simulink model "sampleModel1939"  (R2023a)
settings: Solver=VariableStepAuto  StartTime=0.0  StopTime=10.0  RelTol=1e-3
libraries: hdlsllib x3, simulink x1
settings Model: Creator=user1  LastModifiedBy=user1

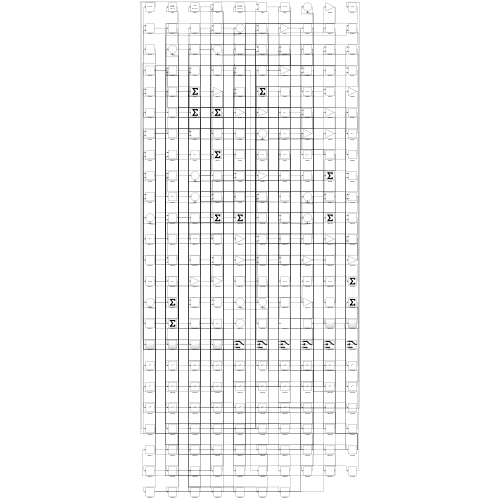
[thumbnail: Simulink's stored preview of the top-level diagram]
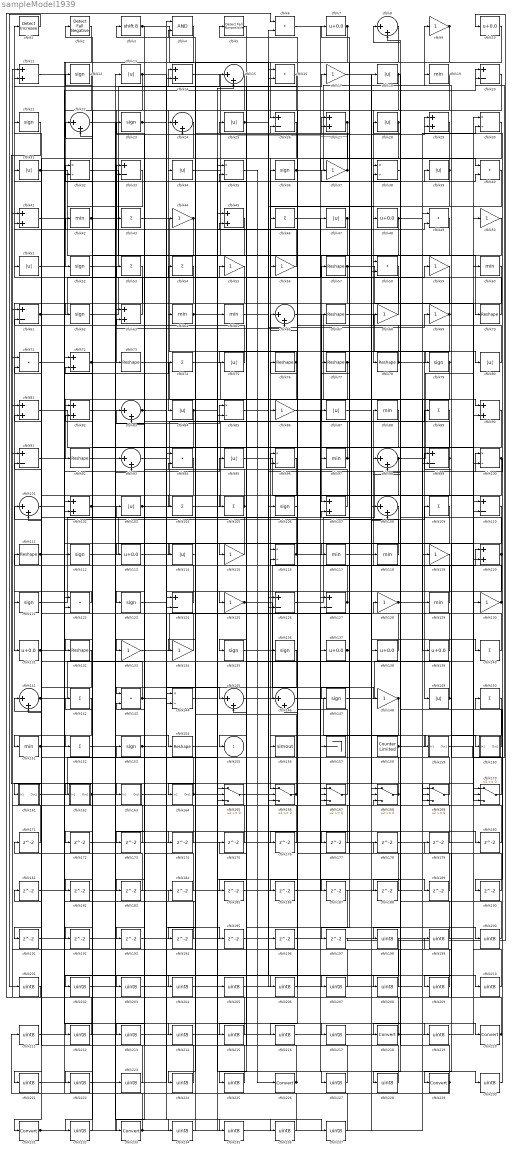
== system sampleModel1939 ==
  cfblk1 : simulink/Logic and Bit Operations/Detect Increase  vinit=0.0  OutDataTypeStr=boolean
      settings: LibrarySourceBlock=|
      | hdlsllib/Logic and Bit
      | Operations/Detect
      | Increase
  cfblk{7,10,48,113,131,137..139} (8 alike) : Bias  Bias=0.0  SaturateOnIntegerOverflow=off
  cfblk{30,32,35,38,85,96,100,116,144} (9 alike) : Product  Inputs=*/  RndMeth=Zero  SaturateOnIntegerOverflow=on
  cfblk{8,15,22,24,66,83,93,98,101,108,141,145..146} (13 alike) : Sum  Inputs=|++
  cfblk{11,14,27,29,41,45,63,72,81..82,90,102,107,120} (14 alike) : Sum
  cfblk{13,18,25,28,31,34,39,47,51,75,80,84,87,95,103,114,149} (17 alike) : Abs  SaturateOnIntegerOverflow=off
  cfblk{43,46,53..54,74,89,104..105,109,140,142,150,152} (13 alike) : Sum  Inputs=+
  cfblk{12,21,23,36,52,62,79,106,112,121,123,135..136,147,153} (15 alike) : Signum
  cfblk{20,26,33,61,91,99,110,124,126..127} (10 alike) : Sum  Inputs=+-
  cfblk{57,67,70,73,76..78,92,111,132,154} (11 alike) : Reshape
  cfblk{9,17,37,44,50,55..56,59,68..69,86,115,119,125,128,130,133..134,148} (19 alike) : Gain
  cfblk{19,42,60,64..65,88,97,117..118,129,151} (11 alike) : MinMax
  cfblk{6,16,40,49,58,71,94,122,143} (9 alike) : DotProduct  OutDataTypeStr=Inherit: Inherit via internal rule
  cfblk156 : ToWorkspace  VariableName=simout  SaveFormat=Timeseries  SampleTime=-1
  cfblk157 : Terminator
  cfblk158 : hdlsllib/Sources/Counter Limited  uplimit=7  tsamp=-1
  cfblk159 : Subsystem
      settings: LibrarySourceBlock=|
      | hdlsllib/Ports &
      | Subsystems/Subsystem
  cfblk160 : Subsystem
      settings: LibrarySourceBlock=|
      | hdlsllib/Ports &
      | Subsystems/Subsystem
  cfblk161 : Subsystem
      settings: LibrarySourceBlock=|
      | hdlsllib/Ports &
      | Subsystems/Subsystem
  cfblk162 : Subsystem
      settings: LibrarySourceBlock=|
      | hdlsllib/Ports &
      | Subsystems/Subsystem
  cfblk163 : Subsystem
      settings: LibrarySourceBlock=|
      | hdlsllib/Ports &
      | Subsystems/Subsystem
  cfblk164 : Subsystem
      settings: LibrarySourceBlock=|
      | hdlsllib/Ports &
      | Subsystems/Subsystem
  cfblk{165..170} (6 alike) : Switch  SaturateOnIntegerOverflow=off  InputSameDT=off
  cfblk{171..197} (27 alike) : Delay  SampleTime=1
  cfblk{198..217,219,221..225,227..228,230,232,234..237} (34 alike) : DataTypeConversion  OutDataTypeStr=uint8  SaturateOnIntegerOverflow=off  RndMeth=Floor
  cfblk2 : hdlsllib/Logic and Bit Operations/Detect Fall Negative  vinit=0  OutDataTypeStr=boolean
  cfblk{218,220,226,229,231,233} (6 alike) : DataTypeConversion  SaturateOnIntegerOverflow=off  RndMeth=Floor
  cfblk3 : ArithShift  BitShiftNumber=8
  cfblk4 : Logic  AllPortsSameDT=off  OutDataTypeStr=boolean
  cfblk5 : hdlsllib/Logic and Bit Operations/Detect Fall Nonpositive  vinit=0  OutDataTypeStr=boolean
  cfblk155 : Outport  VectorParamsAs1DForOutWhenUnconnected=off
  wires:
  cfblk55/1 -> cfblk131/1
  cfblk31/1 -> cfblk70/1, cfblk93/1
  cfblk33/1 -> cfblk73/1
  cfblk121/1 -> cfblk103/1
  cfblk18/1 -> cfblk78/1, cfblk98/2
  cfblk90/1 -> cfblk143/1
  cfblk54/1 -> cfblk233/1
  cfblk47/1 -> cfblk107/1, cfblk62/1
  cfblk57/1 -> cfblk166/1, cfblk100/2
  cfblk78/1 -> cfblk80/1, cfblk5/1
  cfblk126/1 -> cfblk29/1
  cfblk23/1 -> cfblk167/3, cfblk180/1
  cfblk59/1 -> cfblk132/1
  cfblk21/1 -> cfblk163/1(In1)
  cfblk19/1 -> cfblk84/1
  cfblk4/1 -> cfblk52/1
  cfblk25/1 -> cfblk166/2, cfblk48/1, cfblk170/3
  cfblk158/1 -> cfblk160/1(In1), cfblk228/1
  cfblk141/1 -> cfblk18/1, cfblk39/1
  cfblk67/1 -> cfblk149/1
  cfblk26/1 -> cfblk161/1(In1)
  cfblk15/1 -> cfblk152/1
  cfblk28/1 -> cfblk116/1, cfblk165/2
  cfblk145/1 -> cfblk120/1
  cfblk159/1(Out1) -> cfblk20/1
  cfblk43/1 -> cfblk79/1
  cfblk162/1(Out1) -> cfblk85/1, cfblk93/2
  cfblk10/1 -> cfblk125/1
  cfblk130/1 -> cfblk28/1, cfblk32/2
  cfblk68/1 -> cfblk1/1
  cfblk39/1 -> cfblk86/1, cfblk38/1
  cfblk122/1 -> cfblk121/1
  cfblk167/1 -> cfblk14/1
  cfblk37/1 -> cfblk3/1, cfblk24/2, cfblk27/2
  cfblk52/1 -> cfblk17/1
  cfblk111/1 -> cfblk65/1, cfblk20/2
  cfblk75/1 -> cfblk51/1
  cfblk73/1 -> cfblk139/1
  cfblk36/1 -> cfblk9/1, cfblk40/1
  cfblk29/1 -> cfblk34/1
  cfblk41/1 -> cfblk127/1
  cfblk70/1 -> cfblk36/1
  cfblk72/1 -> cfblk232/1, cfblk234/1
  cfblk113/1 -> cfblk115/1
  cfblk84/1 -> cfblk49/2, cfblk222/1
  cfblk69/1 -> cfblk97/1, cfblk2/1
  cfblk143/1 -> cfblk55/1, cfblk111/1
  cfblk66/1 -> cfblk90/1
  cfblk35/1 -> cfblk226/1
  cfblk49/1 -> cfblk155/1
  cfblk80/1 -> cfblk11/2
  cfblk134/1 -> cfblk101/1
  cfblk146/1 -> cfblk159/1(In1)
  cfblk24/1 -> cfblk151/1
  cfblk98/1 -> cfblk60/1, cfblk177/1
  cfblk150/1 -> cfblk229/1
  cfblk104/1 -> cfblk89/1
  cfblk50/1 -> cfblk218/1
  cfblk44/1 -> cfblk182/1, cfblk183/1
  cfblk131/1 -> cfblk72/1, cfblk214/1
  cfblk14/1 -> cfblk146/1
  cfblk30/1 -> cfblk114/1
  cfblk74/1 -> cfblk126/1
  cfblk34/1 -> cfblk157/1
  cfblk9/1 -> cfblk26/1, cfblk185/1
  cfblk46/1 -> cfblk137/1
  cfblk63/1 -> cfblk12/1
  cfblk83/1 -> cfblk44/1, cfblk40/2, cfblk145/1
  cfblk85/1 -> cfblk106/1
  cfblk40/1 -> cfblk156/1
  cfblk148/1 -> cfblk186/1, cfblk187/1
  cfblk169/1 -> cfblk42/1
  cfblk62/1 -> cfblk59/1
  cfblk165/1 -> cfblk100/1
  cfblk151/1 -> cfblk109/1, cfblk74/1
  cfblk117/1 -> cfblk138/1
  cfblk64/1 -> cfblk134/1, cfblk189/1
  cfblk2/1 -> cfblk102/2
  cfblk102/1 -> cfblk154/1, cfblk29/2
  cfblk124/1 -> cfblk61/2
  cfblk76/1 -> cfblk92/1, cfblk75/1
  cfblk170/1 -> cfblk99/1
  cfblk99/1 -> cfblk164/1(In1), cfblk45/2
  cfblk13/1 -> cfblk63/1, cfblk195/1
  cfblk142/1 -> cfblk231/1
  cfblk149/1 -> cfblk15/1, cfblk19/1
  cfblk11/1 -> cfblk112/1
  cfblk17/1 -> cfblk140/1
  cfblk103/1 -> cfblk67/1, cfblk23/1
  cfblk118/1 -> cfblk77/1
  cfblk144/1 -> cfblk220/1
  cfblk97/1 -> cfblk43/1, cfblk197/1
  cfblk105/1 -> cfblk53/1, cfblk83/2
  cfblk153/1 -> cfblk165/3, cfblk236/1
  cfblk32/1 -> cfblk58/1
  cfblk138/1 -> cfblk32/1
  cfblk164/1(Out1) -> cfblk141/1, cfblk227/1
  cfblk27/1 -> cfblk64/1, cfblk133/1
  cfblk137/1 -> cfblk37/1, cfblk7/1
  cfblk161/1(Out1) -> cfblk45/1
  cfblk112/1 -> cfblk87/1
  cfblk107/1 -> cfblk41/2
  cfblk125/1 -> cfblk167/1, cfblk69/1
  cfblk79/1 -> cfblk146/2, cfblk145/2
  cfblk3/1 -> cfblk136/1, cfblk123/1
  cfblk93/1 -> cfblk15/2
  cfblk140/1 -> cfblk76/1
  cfblk127/1 -> cfblk96/1, cfblk25/1
  cfblk168/1 -> cfblk56/1, cfblk27/1
  cfblk115/1 -> cfblk83/1
  cfblk101/1 -> cfblk95/1
  cfblk51/1 -> cfblk120/2
  cfblk53/1 -> cfblk101/2
  cfblk128/1 -> cfblk119/1, cfblk8/2
  cfblk139/1 -> cfblk21/1
  cfblk77/1 -> cfblk147/1, cfblk126/2, cfblk193/1
  cfblk160/1(Out1) -> cfblk68/1
  cfblk56/1 -> cfblk33/1
  cfblk119/1 -> cfblk124/2
  cfblk5/1 -> cfblk105/1
  cfblk120/1 -> cfblk135/1, cfblk116/2, cfblk38/2
  cfblk8/1 -> cfblk117/1
  cfblk95/1 -> cfblk130/1
  cfblk81/1 -> cfblk170/2
  cfblk42/1 -> cfblk66/2, cfblk237/1
  cfblk166/1 -> cfblk4/2, cfblk216/1
  cfblk147/1 -> cfblk30/1
  cfblk92/1 -> cfblk13/1
  cfblk163/1(Out1) -> cfblk57/1
  cfblk129/1 -> cfblk88/1
  cfblk20/1 -> cfblk46/1
  cfblk133/1 -> cfblk118/1
  cfblk87/1 -> cfblk169/3
  cfblk48/1 -> cfblk30/2, cfblk85/2
  cfblk12/1 -> cfblk122/2
  cfblk61/1 -> cfblk47/1, cfblk166/3, cfblk217/1
  cfblk7/1 -> cfblk104/1, cfblk24/1
  cfblk100/1 -> cfblk190/1, cfblk191/1
  cfblk60/1 -> cfblk162/1(In1)
  cfblk109/1 -> cfblk113/1
  cfblk116/1 -> cfblk31/1, cfblk148/1
  cfblk171/1 -> cfblk81/1
  cfblk45/1 -> cfblk172/1
  cfblk172/1 -> cfblk170/1
  cfblk88/1 -> cfblk173/1
  cfblk173/1 -> cfblk41/1
  cfblk152/1 -> cfblk174/1
  cfblk174/1 -> cfblk4/1
  cfblk175/1 -> cfblk124/1
  cfblk106/1 -> cfblk176/1
  cfblk176/1 -> cfblk11/1
  cfblk177/1 -> cfblk72/2
  cfblk179/1 -> cfblk168/3
  cfblk180/1 -> cfblk61/1
  cfblk181/1 -> cfblk169/1
  cfblk182/1 -> cfblk169/2
  cfblk183/1 -> cfblk141/2
  cfblk184/1 -> cfblk143/2
  cfblk185/1 -> cfblk167/2
  cfblk186/1 -> cfblk127/2
  cfblk38/1 -> cfblk188/1
  cfblk188/1 -> cfblk107/2
  cfblk189/1 -> cfblk66/1
  cfblk190/1 -> cfblk96/2
  cfblk191/1 -> cfblk165/1
  cfblk58/1 -> cfblk192/1
  cfblk192/1 -> cfblk90/2
  cfblk193/1 -> cfblk14/2
  cfblk89/1 -> cfblk194/1
  cfblk194/1 -> cfblk122/1
  cfblk195/1 -> cfblk168/2
  cfblk65/1 -> cfblk196/1
  cfblk196/1 -> cfblk99/2
  cfblk197/1 -> cfblk10/1
  cfblk178/1 -> cfblk198/1
  cfblk199/1 -> cfblk178/1
  cfblk6/1 -> cfblk200/1
  cfblk200/1 -> cfblk128/1
  cfblk1/1 -> cfblk201/1
  cfblk201/1 -> cfblk6/1
  cfblk198/1 -> cfblk202/1
  cfblk202/1 -> cfblk6/2
  cfblk16/1 -> cfblk203/1
  cfblk203/1 -> cfblk129/1
  cfblk114/1 -> cfblk204/1
  cfblk204/1 -> cfblk16/1
  cfblk205/1 -> cfblk16/2
  cfblk91/1 -> cfblk206/1
  cfblk206/1 -> cfblk26/2
  cfblk123/1 -> cfblk207/1
  cfblk207/1 -> cfblk91/1
  cfblk71/1 -> cfblk208/1
  cfblk208/1 -> cfblk91/2
  cfblk110/1 -> cfblk209/1
  cfblk209/1 -> cfblk184/1
  cfblk135/1 -> cfblk210/1
  cfblk210/1 -> cfblk110/1
  cfblk211/1 -> cfblk110/2
  cfblk94/1 -> cfblk212/1
  cfblk212/1 -> cfblk181/1
  cfblk136/1 -> cfblk213/1
  cfblk213/1 -> cfblk94/1
  cfblk214/1 -> cfblk94/2
  cfblk108/1 -> cfblk215/1
  cfblk215/1 -> cfblk71/1
  cfblk216/1 -> cfblk108/1
  cfblk217/1 -> cfblk108/2
  cfblk218/1 -> cfblk171/1, cfblk71/2
  cfblk154/1 -> cfblk219/1
  cfblk219/1 -> cfblk50/1
  cfblk220/1 -> cfblk199/1, cfblk179/1, cfblk175/1, cfblk98/1
  cfblk132/1 -> cfblk221/1
  cfblk221/1 -> cfblk144/1
  cfblk222/1 -> cfblk144/2
  cfblk22/1 -> cfblk223/1
  cfblk223/1 -> cfblk81/2
  cfblk96/1 -> cfblk224/1
  cfblk224/1 -> cfblk22/1
  cfblk187/1 -> cfblk225/1
  cfblk225/1 -> cfblk22/2
  cfblk226/1 -> cfblk63/2, cfblk153/1
  cfblk227/1 -> cfblk35/1
  cfblk228/1 -> cfblk35/2
  cfblk229/1 -> cfblk211/1, cfblk8/1
  cfblk86/1 -> cfblk230/1
  cfblk230/1 -> cfblk150/1
  cfblk231/1 -> cfblk58/2, cfblk33/2, cfblk168/1
  cfblk232/1 -> cfblk142/1
  cfblk233/1 -> cfblk205/1, cfblk102/1
  cfblk234/1 -> cfblk54/1
  cfblk82/1 -> cfblk235/1
  cfblk235/1 -> cfblk49/1
  cfblk236/1 -> cfblk82/1
  cfblk237/1 -> cfblk82/2

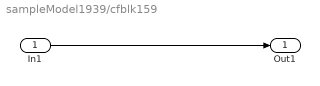
== system sampleModel1939/cfblk159 ==
  In1 : Inport
  Out1 : Outport
  wires:
  In1/1 -> Out1/1

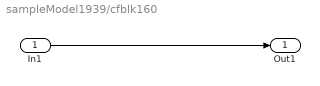
== system sampleModel1939/cfblk160 ==
  In1 : Inport
  Out1 : Outport
  wires:
  In1/1 -> Out1/1

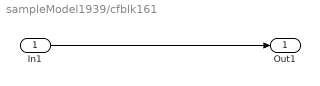
== system sampleModel1939/cfblk161 ==
  In1 : Inport
  Out1 : Outport
  wires:
  In1/1 -> Out1/1

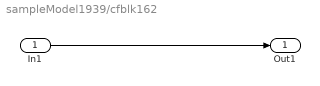
== system sampleModel1939/cfblk162 ==
  In1 : Inport
  Out1 : Outport
  wires:
  In1/1 -> Out1/1

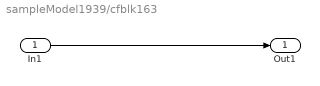
== system sampleModel1939/cfblk163 ==
  In1 : Inport
  Out1 : Outport
  wires:
  In1/1 -> Out1/1

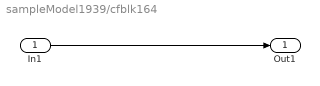
== system sampleModel1939/cfblk164 ==
  In1 : Inport
  Out1 : Outport
  wires:
  In1/1 -> Out1/1
